simulink library "CTRL_UP_SLISUR"  (R2023b)
settings: Solver=VariableStepAuto  StartTime=0.0  StopTime=10.0  RelTol=1e-3
settings Model: Creator=blatak  LastModifiedBy=blatak

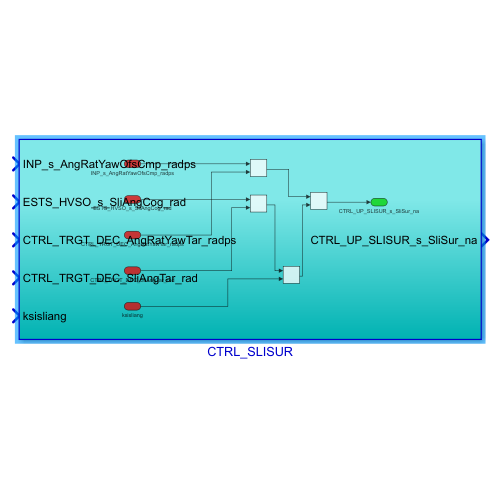
[thumbnail: Simulink's stored preview of the top-level diagram]
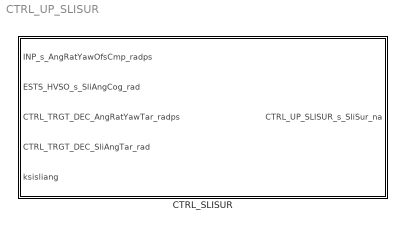
== system CTRL_UP_SLISUR ==
  CTRL_SLISUR : Subsystem

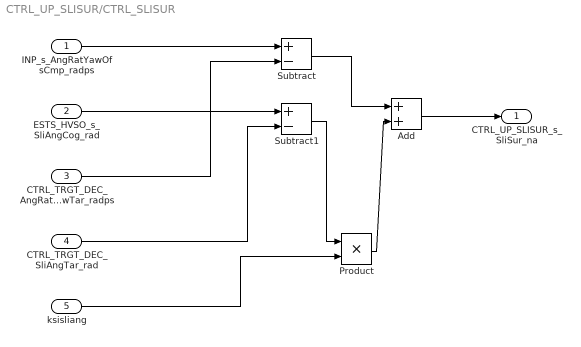
== system CTRL_UP_SLISUR/CTRL_SLISUR ==
  INP_s_AngRatYawOfsCmp_radps : Inport
  ESTS_HVSO_s_SliAngCog_rad : Inport  Port=2
  CTRL_TRGT_DEC_AngRatYawTar_radps : Inport  Port=3
  CTRL_TRGT_DEC_SliAngTar_rad : Inport  Port=4
  ksisliang : Inport  Port=5
  Add : Sum
  Product : Product
  Subtract : Sum  Inputs=+-
  Subtract1 : Sum  Inputs=+-
  CTRL_UP_SLISUR_s_SliSur_na : Outport
  wires:
  Subtract1/1 -> Product/1
  ksisliang/1 -> Product/2
  CTRL_TRGT_DEC_AngRatYawTar_radps/1 -> Subtract/2
  Subtract/1 -> Add/1
  INP_s_AngRatYawOfsCmp_radps/1 -> Subtract/1
  Product/1 -> Add/2
  CTRL_TRGT_DEC_SliAngTar_rad/1 -> Subtract1/2
  ESTS_HVSO_s_SliAngCog_rad/1 -> Subtract1/1
  Add/1 -> CTRL_UP_SLISUR_s_SliSur_na/1
